simulink model "vit_tiny_simulink"  (R2026a)
settings: Solver=FixedStepAuto
values from neighbouring files (symbols this model uses):
  quantNet = quantize(quantObj)    [quantize_network.m]
libraries: dlconvfclib x26, dlnormalizationlib x25, dlcombinationlib x24, dlactivationlib x12
settings Model: Creator=arkadiyturevskiy  LastModifiedBy=arkadiyturevskiy
settings HardwareCC: ProdLargestAtomicInteger=Long  ProdLargestAtomicFloat=Double  ProdHWDeviceType=ARM Compatible->ARM Cortex-A
settings RTWCC: SystemTargetFile=ert.tlc  GenCodeOnly=on  GenerateReport=on  Description=Embedded Coder
settings ERTTargetCC: GenerateSampleERTMain=on

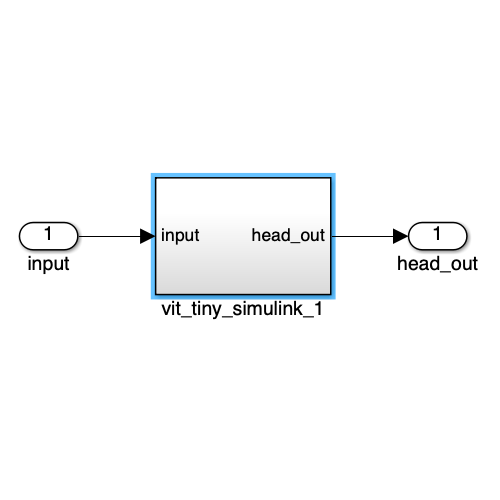
[thumbnail: Simulink's stored preview of the top-level diagram]
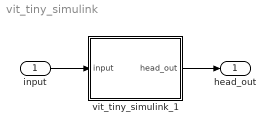
== system vit_tiny_simulink ==
  input : Inport  OutDataTypeStr=single  PortDimensions="[224  224    3]"
  vit_tiny_simulink_1 : Subsystem
  head_out : Outport
  wires:
  vit_tiny_simulink_1/1(head_out) -> head_out/1
  input/1 -> vit_tiny_simulink_1/1(input)

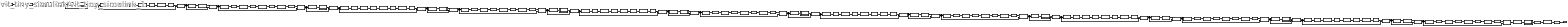
== system vit_tiny_simulink/vit_tiny_simulink_1 ==
  input : Inport  OutDataTypeStr=single  PortDimensions="[224  224    3]"
  block0_add1 : dlcombinationlib/Addition Layer  NumInputs=2  OutMin=[]  OutMax=[]  InternalRndMeth=Floor  InternalSaturateOnIntegerOverflow=off  SampleTime=-1
      settings: DataFormat=CT
  block0_add2 : dlcombinationlib/Addition Layer  NumInputs=2  OutMin=[]  OutMax=[]  InternalRndMeth=Floor  InternalSaturateOnIntegerOverflow=off  SampleTime=-1
      settings: DataFormat=CT
  block0_attn : Subsystem
  block0_fc1 : dlconvfclib/Fully Connected Layer  Layer=quantNet.Layers(10)  OutMin=[]  OutMax=[]  OutDataTypeStr=fixdt(1,32,9)  RndMeth=Nearest  WeightsDataTypeStr=fixdt(1,8,7)  WeightsMin=[]  WeightsMax=[]  BiasDataTypeStr=fixdt(1,32,9)  BiasMin=[]  BiasMax=[]  AccumDataTypeStr=fixdt(1,32,9)  AccumMin=[]  AccumMax=[]  InternalRndMeth=Nearest  InternalSaturateOnIntegerOverflow=off  SampleTime=-1
      settings: DataFormat=CT
  block0_fc1_in_cast : DataTypeConversion  OutDataTypeStr=fixdt(1,8,2)  RndMeth=Nearest
  block0_fc1_out_cast : DataTypeConversion  OutDataTypeStr=fixdt('single')  RndMeth=Nearest
  block0_fc2 : dlconvfclib/Fully Connected Layer  Layer=quantNet.Layers(12)  OutMin=[]  OutMax=[]  OutDataTypeStr=fixdt(1,32,9)  RndMeth=Nearest  WeightsDataTypeStr=fixdt(1,8,7)  WeightsMin=[]  WeightsMax=[]  BiasDataTypeStr=fixdt(1,32,9)  BiasMin=[]  BiasMax=[]  AccumDataTypeStr=fixdt(1,32,9)  AccumMin=[]  AccumMax=[]  InternalRndMeth=Nearest  InternalSaturateOnIntegerOverflow=off  SampleTime=-1
      settings: DataFormat=CT
  block0_fc2_in_cast : DataTypeConversion  OutDataTypeStr=fixdt(1,8,2)  RndMeth=Nearest
  block0_fc2_out_cast : DataTypeConversion  OutDataTypeStr=fixdt('single')  RndMeth=Nearest
  block0_gelu : dlactivationlib/GELU Layer  Approximation=none  OutMin=[]  OutMax=[]  SampleTime=-1
  block0_ln1 : dlnormalizationlib/Layer Normalization Layer  Layer=quantNet.Layers(6)  OutMin=[]  OutMax=[]  ScaleDataTypeStr=Inherit: Inherit via back propagation  ScaleMin=[]  ScaleMax=[]  OffsetDataTypeStr=Inherit: Inherit via back propagation  OffsetMin=[]  OffsetMax=[]  SampleTime=-1
      settings: DataFormat=CT
  block0_ln2 : dlnormalizationlib/Layer Normalization Layer  Layer=quantNet.Layers(9)  OutMin=[]  OutMax=[]  ScaleDataTypeStr=Inherit: Inherit via back propagation  ScaleMin=[]  ScaleMax=[]  OffsetDataTypeStr=Inherit: Inherit via back propagation  OffsetMin=[]  OffsetMax=[]  SampleTime=-1
      settings: DataFormat=CT
  block10_add1 : dlcombinationlib/Addition Layer  NumInputs=2  OutMin=[]  OutMax=[]  InternalRndMeth=Floor  InternalSaturateOnIntegerOverflow=off  SampleTime=-1
      settings: DataFormat=CT
  block10_add2 : dlcombinationlib/Addition Layer  NumInputs=2  OutMin=[]  OutMax=[]  InternalRndMeth=Floor  InternalSaturateOnIntegerOverflow=off  SampleTime=-1
      settings: DataFormat=CT
  block10_attn : Subsystem
  block10_fc1 : dlconvfclib/Fully Connected Layer  Layer=quantNet.Layers(90)  OutMin=[]  OutMax=[]  OutDataTypeStr=fixdt(1,32,10)  RndMeth=Nearest  WeightsDataTypeStr=fixdt(1,8,7)  WeightsMin=[]  WeightsMax=[]  BiasDataTypeStr=fixdt(1,32,10)  BiasMin=[]  BiasMax=[]  AccumDataTypeStr=fixdt(1,32,10)  AccumMin=[]  AccumMax=[]  InternalRndMeth=Nearest  InternalSaturateOnIntegerOverflow=off  SampleTime=-1
      settings: DataFormat=CT
  block10_fc1_in_cast : DataTypeConversion  OutDataTypeStr=fixdt(1,8,3)  RndMeth=Nearest
  block10_fc1_out_cast : DataTypeConversion  OutDataTypeStr=fixdt('single')  RndMeth=Nearest
  block10_fc2 : dlconvfclib/Fully Connected Layer  Layer=quantNet.Layers(92)  OutMin=[]  OutMax=[]  OutDataTypeStr=fixdt(1,32,11)  RndMeth=Nearest  WeightsDataTypeStr=fixdt(1,8,7)  WeightsMin=[]  WeightsMax=[]  BiasDataTypeStr=fixdt(1,32,11)  BiasMin=[]  BiasMax=[]  AccumDataTypeStr=fixdt(1,32,11)  AccumMin=[]  AccumMax=[]  InternalRndMeth=Nearest  InternalSaturateOnIntegerOverflow=off  SampleTime=-1
      settings: DataFormat=CT
  block10_fc2_in_cast : DataTypeConversion  OutDataTypeStr=fixdt(1,8,4)  RndMeth=Nearest
  block10_fc2_out_cast : DataTypeConversion  OutDataTypeStr=fixdt('single')  RndMeth=Nearest
  block10_gelu : dlactivationlib/GELU Layer  Approximation=none  OutMin=[]  OutMax=[]  SampleTime=-1
  block10_ln1 : dlnormalizationlib/Layer Normalization Layer  Layer=quantNet.Layers(86)  OutMin=[]  OutMax=[]  ScaleDataTypeStr=Inherit: Inherit via back propagation  ScaleMin=[]  ScaleMax=[]  OffsetDataTypeStr=Inherit: Inherit via back propagation  OffsetMin=[]  OffsetMax=[]  SampleTime=-1
      settings: DataFormat=CT
  block10_ln2 : dlnormalizationlib/Layer Normalization Layer  Layer=quantNet.Layers(89)  OutMin=[]  OutMax=[]  ScaleDataTypeStr=Inherit: Inherit via back propagation  ScaleMin=[]  ScaleMax=[]  OffsetDataTypeStr=Inherit: Inherit via back propagation  OffsetMin=[]  OffsetMax=[]  SampleTime=-1
      settings: DataFormat=CT
  block11_add1 : dlcombinationlib/Addition Layer  NumInputs=2  OutMin=[]  OutMax=[]  InternalRndMeth=Floor  InternalSaturateOnIntegerOverflow=off  SampleTime=-1
      settings: DataFormat=CT
  block11_add2 : dlcombinationlib/Addition Layer  NumInputs=2  OutMin=[]  OutMax=[]  InternalRndMeth=Floor  InternalSaturateOnIntegerOverflow=off  SampleTime=-1
      settings: DataFormat=CT
  block11_attn : Subsystem
  block11_fc1 : dlconvfclib/Fully Connected Layer  Layer=quantNet.Layers(98)  OutMin=[]  OutMax=[]  OutDataTypeStr=fixdt(1,32,11)  RndMeth=Nearest  WeightsDataTypeStr=fixdt(1,8,8)  WeightsMin=[]  WeightsMax=[]  BiasDataTypeStr=fixdt(1,32,11)  BiasMin=[]  BiasMax=[]  AccumDataTypeStr=fixdt(1,32,11)  AccumMin=[]  AccumMax=[]  InternalRndMeth=Nearest  InternalSaturateOnIntegerOverflow=off  SampleTime=-1
      settings: DataFormat=CT
  block11_fc1_in_cast : DataTypeConversion  OutDataTypeStr=fixdt(1,8,3)  RndMeth=Nearest
  block11_fc1_out_cast : DataTypeConversion  OutDataTypeStr=fixdt('single')  RndMeth=Nearest
  block11_fc2 : dlconvfclib/Fully Connected Layer  Layer=quantNet.Layers(100)  OutMin=[]  OutMax=[]  OutDataTypeStr=fixdt(1,32,11)  RndMeth=Nearest  WeightsDataTypeStr=fixdt(1,8,7)  WeightsMin=[]  WeightsMax=[]  BiasDataTypeStr=fixdt(1,32,11)  BiasMin=[]  BiasMax=[]  AccumDataTypeStr=fixdt(1,32,11)  AccumMin=[]  AccumMax=[]  InternalRndMeth=Nearest  InternalSaturateOnIntegerOverflow=off  SampleTime=-1
      settings: DataFormat=CT
  block11_fc2_in_cast : DataTypeConversion  OutDataTypeStr=fixdt(1,8,4)  RndMeth=Nearest
  block11_fc2_out_cast : DataTypeConversion  OutDataTypeStr=fixdt('single')  RndMeth=Nearest
  block11_gelu : dlactivationlib/GELU Layer  Approximation=none  OutMin=[]  OutMax=[]  SampleTime=-1
  block11_ln1 : dlnormalizationlib/Layer Normalization Layer  Layer=quantNet.Layers(94)  OutMin=[]  OutMax=[]  ScaleDataTypeStr=Inherit: Inherit via back propagation  ScaleMin=[]  ScaleMax=[]  OffsetDataTypeStr=Inherit: Inherit via back propagation  OffsetMin=[]  OffsetMax=[]  SampleTime=-1
      settings: DataFormat=CT
  block11_ln2 : dlnormalizationlib/Layer Normalization Layer  Layer=quantNet.Layers(97)  OutMin=[]  OutMax=[]  ScaleDataTypeStr=Inherit: Inherit via back propagation  ScaleMin=[]  ScaleMax=[]  OffsetDataTypeStr=Inherit: Inherit via back propagation  OffsetMin=[]  OffsetMax=[]  SampleTime=-1
      settings: DataFormat=CT
  block1_add1 : dlcombinationlib/Addition Layer  NumInputs=2  OutMin=[]  OutMax=[]  InternalRndMeth=Floor  InternalSaturateOnIntegerOverflow=off  SampleTime=-1
      settings: DataFormat=CT
  block1_add2 : dlcombinationlib/Addition Layer  NumInputs=2  OutMin=[]  OutMax=[]  InternalRndMeth=Floor  InternalSaturateOnIntegerOverflow=off  SampleTime=-1
      settings: DataFormat=CT
  block1_attn : Subsystem
  block1_fc1 : dlconvfclib/Fully Connected Layer  Layer=quantNet.Layers(18)  OutMin=[]  OutMax=[]  OutDataTypeStr=fixdt(1,32,10)  RndMeth=Nearest  WeightsDataTypeStr=fixdt(1,8,7)  WeightsMin=[]  WeightsMax=[]  BiasDataTypeStr=fixdt(1,32,10)  BiasMin=[]  BiasMax=[]  AccumDataTypeStr=fixdt(1,32,10)  AccumMin=[]  AccumMax=[]  InternalRndMeth=Nearest  InternalSaturateOnIntegerOverflow=off  SampleTime=-1
      settings: DataFormat=CT
  block1_fc1_in_cast : DataTypeConversion  OutDataTypeStr=fixdt(1,8,3)  RndMeth=Nearest
  block1_fc1_out_cast : DataTypeConversion  OutDataTypeStr=fixdt('single')  RndMeth=Nearest
  block1_fc2 : dlconvfclib/Fully Connected Layer  Layer=quantNet.Layers(20)  OutMin=[]  OutMax=[]  OutDataTypeStr=fixdt(1,32,10)  RndMeth=Nearest  WeightsDataTypeStr=fixdt(1,8,7)  WeightsMin=[]  WeightsMax=[]  BiasDataTypeStr=fixdt(1,32,10)  BiasMin=[]  BiasMax=[]  AccumDataTypeStr=fixdt(1,32,10)  AccumMin=[]  AccumMax=[]  InternalRndMeth=Nearest  InternalSaturateOnIntegerOverflow=off  SampleTime=-1
      settings: DataFormat=CT
  block1_fc2_in_cast : DataTypeConversion  OutDataTypeStr=fixdt(1,8,3)  RndMeth=Nearest
  block1_fc2_out_cast : DataTypeConversion  OutDataTypeStr=fixdt('single')  RndMeth=Nearest
  block1_gelu : dlactivationlib/GELU Layer  Approximation=none  OutMin=[]  OutMax=[]  SampleTime=-1
  block1_ln1 : dlnormalizationlib/Layer Normalization Layer  Layer=quantNet.Layers(14)  OutMin=[]  OutMax=[]  ScaleDataTypeStr=Inherit: Inherit via back propagation  ScaleMin=[]  ScaleMax=[]  OffsetDataTypeStr=Inherit: Inherit via back propagation  OffsetMin=[]  OffsetMax=[]  SampleTime=-1
      settings: DataFormat=CT
  block1_ln2 : dlnormalizationlib/Layer Normalization Layer  Layer=quantNet.Layers(17)  OutMin=[]  OutMax=[]  ScaleDataTypeStr=Inherit: Inherit via back propagation  ScaleMin=[]  ScaleMax=[]  OffsetDataTypeStr=Inherit: Inherit via back propagation  OffsetMin=[]  OffsetMax=[]  SampleTime=-1
      settings: DataFormat=CT
  block2_add1 : dlcombinationlib/Addition Layer  NumInputs=2  OutMin=[]  OutMax=[]  InternalRndMeth=Floor  InternalSaturateOnIntegerOverflow=off  SampleTime=-1
      settings: DataFormat=CT
  block2_add2 : dlcombinationlib/Addition Layer  NumInputs=2  OutMin=[]  OutMax=[]  InternalRndMeth=Floor  InternalSaturateOnIntegerOverflow=off  SampleTime=-1
      settings: DataFormat=CT
  block2_attn : Subsystem
  block2_fc1 : dlconvfclib/Fully Connected Layer  Layer=quantNet.Layers(26)  OutMin=[]  OutMax=[]  OutDataTypeStr=fixdt(1,32,10)  RndMeth=Nearest  WeightsDataTypeStr=fixdt(1,8,7)  WeightsMin=[]  WeightsMax=[]  BiasDataTypeStr=fixdt(1,32,10)  BiasMin=[]  BiasMax=[]  AccumDataTypeStr=fixdt(1,32,10)  AccumMin=[]  AccumMax=[]  InternalRndMeth=Nearest  InternalSaturateOnIntegerOverflow=off  SampleTime=-1
      settings: DataFormat=CT
  block2_fc1_in_cast : DataTypeConversion  OutDataTypeStr=fixdt(1,8,3)  RndMeth=Nearest
  block2_fc1_out_cast : DataTypeConversion  OutDataTypeStr=fixdt('single')  RndMeth=Nearest
  block2_fc2 : dlconvfclib/Fully Connected Layer  Layer=quantNet.Layers(28)  OutMin=[]  OutMax=[]  OutDataTypeStr=fixdt(1,32,10)  RndMeth=Nearest  WeightsDataTypeStr=fixdt(1,8,7)  WeightsMin=[]  WeightsMax=[]  BiasDataTypeStr=fixdt(1,32,10)  BiasMin=[]  BiasMax=[]  AccumDataTypeStr=fixdt(1,32,10)  AccumMin=[]  AccumMax=[]  InternalRndMeth=Nearest  InternalSaturateOnIntegerOverflow=off  SampleTime=-1
      settings: DataFormat=CT
  block2_fc2_in_cast : DataTypeConversion  OutDataTypeStr=fixdt(1,8,3)  RndMeth=Nearest
  block2_fc2_out_cast : DataTypeConversion  OutDataTypeStr=fixdt('single')  RndMeth=Nearest
  block2_gelu : dlactivationlib/GELU Layer  Approximation=none  OutMin=[]  OutMax=[]  SampleTime=-1
  block2_ln1 : dlnormalizationlib/Layer Normalization Layer  Layer=quantNet.Layers(22)  OutMin=[]  OutMax=[]  ScaleDataTypeStr=Inherit: Inherit via back propagation  ScaleMin=[]  ScaleMax=[]  OffsetDataTypeStr=Inherit: Inherit via back propagation  OffsetMin=[]  OffsetMax=[]  SampleTime=-1
      settings: DataFormat=CT
  block2_ln2 : dlnormalizationlib/Layer Normalization Layer  Layer=quantNet.Layers(25)  OutMin=[]  OutMax=[]  ScaleDataTypeStr=Inherit: Inherit via back propagation  ScaleMin=[]  ScaleMax=[]  OffsetDataTypeStr=Inherit: Inherit via back propagation  OffsetMin=[]  OffsetMax=[]  SampleTime=-1
      settings: DataFormat=CT
  block3_add1 : dlcombinationlib/Addition Layer  NumInputs=2  OutMin=[]  OutMax=[]  InternalRndMeth=Floor  InternalSaturateOnIntegerOverflow=off  SampleTime=-1
      settings: DataFormat=CT
  block3_add2 : dlcombinationlib/Addition Layer  NumInputs=2  OutMin=[]  OutMax=[]  InternalRndMeth=Floor  InternalSaturateOnIntegerOverflow=off  SampleTime=-1
      settings: DataFormat=CT
  block3_attn : Subsystem
  block3_fc1 : dlconvfclib/Fully Connected Layer  Layer=quantNet.Layers(34)  OutMin=[]  OutMax=[]  OutDataTypeStr=fixdt(1,32,10)  RndMeth=Nearest  WeightsDataTypeStr=fixdt(1,8,7)  WeightsMin=[]  WeightsMax=[]  BiasDataTypeStr=fixdt(1,32,10)  BiasMin=[]  BiasMax=[]  AccumDataTypeStr=fixdt(1,32,10)  AccumMin=[]  AccumMax=[]  InternalRndMeth=Nearest  InternalSaturateOnIntegerOverflow=off  SampleTime=-1
      settings: DataFormat=CT
  block3_fc1_in_cast : DataTypeConversion  OutDataTypeStr=fixdt(1,8,3)  RndMeth=Nearest
  block3_fc1_out_cast : DataTypeConversion  OutDataTypeStr=fixdt('single')  RndMeth=Nearest
  block3_fc2 : dlconvfclib/Fully Connected Layer  Layer=quantNet.Layers(36)  OutMin=[]  OutMax=[]  OutDataTypeStr=fixdt(1,32,11)  RndMeth=Nearest  WeightsDataTypeStr=fixdt(1,8,7)  WeightsMin=[]  WeightsMax=[]  BiasDataTypeStr=fixdt(1,32,11)  BiasMin=[]  BiasMax=[]  AccumDataTypeStr=fixdt(1,32,11)  AccumMin=[]  AccumMax=[]  InternalRndMeth=Nearest  InternalSaturateOnIntegerOverflow=off  SampleTime=-1
      settings: DataFormat=CT
  block3_fc2_in_cast : DataTypeConversion  OutDataTypeStr=fixdt(1,8,4)  RndMeth=Nearest
  block3_fc2_out_cast : DataTypeConversion  OutDataTypeStr=fixdt('single')  RndMeth=Nearest
  block3_gelu : dlactivationlib/GELU Layer  Approximation=none  OutMin=[]  OutMax=[]  SampleTime=-1
  block3_ln1 : dlnormalizationlib/Layer Normalization Layer  Layer=quantNet.Layers(30)  OutMin=[]  OutMax=[]  ScaleDataTypeStr=Inherit: Inherit via back propagation  ScaleMin=[]  ScaleMax=[]  OffsetDataTypeStr=Inherit: Inherit via back propagation  OffsetMin=[]  OffsetMax=[]  SampleTime=-1
      settings: DataFormat=CT
  block3_ln2 : dlnormalizationlib/Layer Normalization Layer  Layer=quantNet.Layers(33)  OutMin=[]  OutMax=[]  ScaleDataTypeStr=Inherit: Inherit via back propagation  ScaleMin=[]  ScaleMax=[]  OffsetDataTypeStr=Inherit: Inherit via back propagation  OffsetMin=[]  OffsetMax=[]  SampleTime=-1
      settings: DataFormat=CT
  block4_add1 : dlcombinationlib/Addition Layer  NumInputs=2  OutMin=[]  OutMax=[]  InternalRndMeth=Floor  InternalSaturateOnIntegerOverflow=off  SampleTime=-1
      settings: DataFormat=CT
  block4_add2 : dlcombinationlib/Addition Layer  NumInputs=2  OutMin=[]  OutMax=[]  InternalRndMeth=Floor  InternalSaturateOnIntegerOverflow=off  SampleTime=-1
      settings: DataFormat=CT
  block4_attn : Subsystem
  block4_fc1 : dlconvfclib/Fully Connected Layer  Layer=quantNet.Layers(42)  OutMin=[]  OutMax=[]  OutDataTypeStr=fixdt(1,32,12)  RndMeth=Nearest  WeightsDataTypeStr=fixdt(1,8,8)  WeightsMin=[]  WeightsMax=[]  BiasDataTypeStr=fixdt(1,32,12)  BiasMin=[]  BiasMax=[]  AccumDataTypeStr=fixdt(1,32,12)  AccumMin=[]  AccumMax=[]  InternalRndMeth=Nearest  InternalSaturateOnIntegerOverflow=off  SampleTime=-1
      settings: DataFormat=CT
  block4_fc1_in_cast : DataTypeConversion  OutDataTypeStr=fixdt(1,8,4)  RndMeth=Nearest
  block4_fc1_out_cast : DataTypeConversion  OutDataTypeStr=fixdt('single')  RndMeth=Nearest
  block4_fc2 : dlconvfclib/Fully Connected Layer  Layer=quantNet.Layers(44)  OutMin=[]  OutMax=[]  OutDataTypeStr=fixdt(1,32,12)  RndMeth=Nearest  WeightsDataTypeStr=fixdt(1,8,8)  WeightsMin=[]  WeightsMax=[]  BiasDataTypeStr=fixdt(1,32,12)  BiasMin=[]  BiasMax=[]  AccumDataTypeStr=fixdt(1,32,12)  AccumMin=[]  AccumMax=[]  InternalRndMeth=Nearest  InternalSaturateOnIntegerOverflow=off  SampleTime=-1
      settings: DataFormat=CT
  block4_fc2_in_cast : DataTypeConversion  OutDataTypeStr=fixdt(1,8,4)  RndMeth=Nearest
  block4_fc2_out_cast : DataTypeConversion  OutDataTypeStr=fixdt('single')  RndMeth=Nearest
  block4_gelu : dlactivationlib/GELU Layer  Approximation=none  OutMin=[]  OutMax=[]  SampleTime=-1
  block4_ln1 : dlnormalizationlib/Layer Normalization Layer  Layer=quantNet.Layers(38)  OutMin=[]  OutMax=[]  ScaleDataTypeStr=Inherit: Inherit via back propagation  ScaleMin=[]  ScaleMax=[]  OffsetDataTypeStr=Inherit: Inherit via back propagation  OffsetMin=[]  OffsetMax=[]  SampleTime=-1
      settings: DataFormat=CT
  block4_ln2 : dlnormalizationlib/Layer Normalization Layer  Layer=quantNet.Layers(41)  OutMin=[]  OutMax=[]  ScaleDataTypeStr=Inherit: Inherit via back propagation  ScaleMin=[]  ScaleMax=[]  OffsetDataTypeStr=Inherit: Inherit via back propagation  OffsetMin=[]  OffsetMax=[]  SampleTime=-1
      settings: DataFormat=CT
  block5_add1 : dlcombinationlib/Addition Layer  NumInputs=2  OutMin=[]  OutMax=[]  InternalRndMeth=Floor  InternalSaturateOnIntegerOverflow=off  SampleTime=-1
      settings: DataFormat=CT
  block5_add2 : dlcombinationlib/Addition Layer  NumInputs=2  OutMin=[]  OutMax=[]  InternalRndMeth=Floor  InternalSaturateOnIntegerOverflow=off  SampleTime=-1
      settings: DataFormat=CT
  block5_attn : Subsystem
  block5_fc1 : dlconvfclib/Fully Connected Layer  Layer=quantNet.Layers(50)  OutMin=[]  OutMax=[]  OutDataTypeStr=fixdt(1,32,12)  RndMeth=Nearest  WeightsDataTypeStr=fixdt(1,8,8)  WeightsMin=[]  WeightsMax=[]  BiasDataTypeStr=fixdt(1,32,12)  BiasMin=[]  BiasMax=[]  AccumDataTypeStr=fixdt(1,32,12)  AccumMin=[]  AccumMax=[]  InternalRndMeth=Nearest  InternalSaturateOnIntegerOverflow=off  SampleTime=-1
      settings: DataFormat=CT
  block5_fc1_in_cast : DataTypeConversion  OutDataTypeStr=fixdt(1,8,4)  RndMeth=Nearest
  block5_fc1_out_cast : DataTypeConversion  OutDataTypeStr=fixdt('single')  RndMeth=Nearest
  block5_fc2 : dlconvfclib/Fully Connected Layer  Layer=quantNet.Layers(52)  OutMin=[]  OutMax=[]  OutDataTypeStr=fixdt(1,32,12)  RndMeth=Nearest  WeightsDataTypeStr=fixdt(1,8,8)  WeightsMin=[]  WeightsMax=[]  BiasDataTypeStr=fixdt(1,32,12)  BiasMin=[]  BiasMax=[]  AccumDataTypeStr=fixdt(1,32,12)  AccumMin=[]  AccumMax=[]  InternalRndMeth=Nearest  InternalSaturateOnIntegerOverflow=off  SampleTime=-1
      settings: DataFormat=CT
  block5_fc2_in_cast : DataTypeConversion  OutDataTypeStr=fixdt(1,8,4)  RndMeth=Nearest
  block5_fc2_out_cast : DataTypeConversion  OutDataTypeStr=fixdt('single')  RndMeth=Nearest
  block5_gelu : dlactivationlib/GELU Layer  Approximation=none  OutMin=[]  OutMax=[]  SampleTime=-1
  block5_ln1 : dlnormalizationlib/Layer Normalization Layer  Layer=quantNet.Layers(46)  OutMin=[]  OutMax=[]  ScaleDataTypeStr=Inherit: Inherit via back propagation  ScaleMin=[]  ScaleMax=[]  OffsetDataTypeStr=Inherit: Inherit via back propagation  OffsetMin=[]  OffsetMax=[]  SampleTime=-1
      settings: DataFormat=CT
  block5_ln2 : dlnormalizationlib/Layer Normalization Layer  Layer=quantNet.Layers(49)  OutMin=[]  OutMax=[]  ScaleDataTypeStr=Inherit: Inherit via back propagation  ScaleMin=[]  ScaleMax=[]  OffsetDataTypeStr=Inherit: Inherit via back propagation  OffsetMin=[]  OffsetMax=[]  SampleTime=-1
      settings: DataFormat=CT
  block6_add1 : dlcombinationlib/Addition Layer  NumInputs=2  OutMin=[]  OutMax=[]  InternalRndMeth=Floor  InternalSaturateOnIntegerOverflow=off  SampleTime=-1
      settings: DataFormat=CT
  block6_add2 : dlcombinationlib/Addition Layer  NumInputs=2  OutMin=[]  OutMax=[]  InternalRndMeth=Floor  InternalSaturateOnIntegerOverflow=off  SampleTime=-1
      settings: DataFormat=CT
  block6_attn : Subsystem
  block6_fc1 : dlconvfclib/Fully Connected Layer  Layer=quantNet.Layers(58)  OutMin=[]  OutMax=[]  OutDataTypeStr=fixdt(1,32,12)  RndMeth=Nearest  WeightsDataTypeStr=fixdt(1,8,8)  WeightsMin=[]  WeightsMax=[]  BiasDataTypeStr=fixdt(1,32,12)  BiasMin=[]  BiasMax=[]  AccumDataTypeStr=fixdt(1,32,12)  AccumMin=[]  AccumMax=[]  InternalRndMeth=Nearest  InternalSaturateOnIntegerOverflow=off  SampleTime=-1
      settings: DataFormat=CT
  block6_fc1_in_cast : DataTypeConversion  OutDataTypeStr=fixdt(1,8,4)  RndMeth=Nearest
  block6_fc1_out_cast : DataTypeConversion  OutDataTypeStr=fixdt('single')  RndMeth=Nearest
  block6_fc2 : dlconvfclib/Fully Connected Layer  Layer=quantNet.Layers(60)  OutMin=[]  OutMax=[]  OutDataTypeStr=fixdt(1,32,10)  RndMeth=Nearest  WeightsDataTypeStr=fixdt(1,8,7)  WeightsMin=[]  WeightsMax=[]  BiasDataTypeStr=fixdt(1,32,10)  BiasMin=[]  BiasMax=[]  AccumDataTypeStr=fixdt(1,32,10)  AccumMin=[]  AccumMax=[]  InternalRndMeth=Nearest  InternalSaturateOnIntegerOverflow=off  SampleTime=-1
      settings: DataFormat=CT
  block6_fc2_in_cast : DataTypeConversion  OutDataTypeStr=fixdt(1,8,3)  RndMeth=Nearest
  block6_fc2_out_cast : DataTypeConversion  OutDataTypeStr=fixdt('single')  RndMeth=Nearest
  block6_gelu : dlactivationlib/GELU Layer  Approximation=none  OutMin=[]  OutMax=[]  SampleTime=-1
  block6_ln1 : dlnormalizationlib/Layer Normalization Layer  Layer=quantNet.Layers(54)  OutMin=[]  OutMax=[]  ScaleDataTypeStr=Inherit: Inherit via back propagation  ScaleMin=[]  ScaleMax=[]  OffsetDataTypeStr=Inherit: Inherit via back propagation  OffsetMin=[]  OffsetMax=[]  SampleTime=-1
      settings: DataFormat=CT
  block6_ln2 : dlnormalizationlib/Layer Normalization Layer  Layer=quantNet.Layers(57)  OutMin=[]  OutMax=[]  ScaleDataTypeStr=Inherit: Inherit via back propagation  ScaleMin=[]  ScaleMax=[]  OffsetDataTypeStr=Inherit: Inherit via back propagation  OffsetMin=[]  OffsetMax=[]  SampleTime=-1
      settings: DataFormat=CT
  block7_add1 : dlcombinationlib/Addition Layer  NumInputs=2  OutMin=[]  OutMax=[]  InternalRndMeth=Floor  InternalSaturateOnIntegerOverflow=off  SampleTime=-1
      settings: DataFormat=CT
  block7_add2 : dlcombinationlib/Addition Layer  NumInputs=2  OutMin=[]  OutMax=[]  InternalRndMeth=Floor  InternalSaturateOnIntegerOverflow=off  SampleTime=-1
      settings: DataFormat=CT
  block7_attn : Subsystem
  block7_fc1 : dlconvfclib/Fully Connected Layer  Layer=quantNet.Layers(66)  OutMin=[]  OutMax=[]  OutDataTypeStr=fixdt(1,32,9)  RndMeth=Nearest  WeightsDataTypeStr=fixdt(1,8,5)  WeightsMin=[]  WeightsMax=[]  BiasDataTypeStr=fixdt(1,32,9)  BiasMin=[]  BiasMax=[]  AccumDataTypeStr=fixdt(1,32,9)  AccumMin=[]  AccumMax=[]  InternalRndMeth=Nearest  InternalSaturateOnIntegerOverflow=off  SampleTime=-1
      settings: DataFormat=CT
  block7_fc1_in_cast : DataTypeConversion  OutDataTypeStr=fixdt(1,8,4)  RndMeth=Nearest
  block7_fc1_out_cast : DataTypeConversion  OutDataTypeStr=fixdt('single')  RndMeth=Nearest
  block7_fc2 : dlconvfclib/Fully Connected Layer  Layer=quantNet.Layers(68)  OutMin=[]  OutMax=[]  OutDataTypeStr=fixdt(1,32,4)  RndMeth=Nearest  WeightsDataTypeStr=fixdt(1,8,5)  WeightsMin=[]  WeightsMax=[]  BiasDataTypeStr=fixdt(1,32,4)  BiasMin=[]  BiasMax=[]  AccumDataTypeStr=fixdt(1,32,4)  AccumMin=[]  AccumMax=[]  InternalRndMeth=Nearest  InternalSaturateOnIntegerOverflow=off  SampleTime=-1
      settings: DataFormat=CT
  block7_fc2_in_cast : DataTypeConversion  OutDataTypeStr=fixdt(1,8,-1)  RndMeth=Nearest
  block7_fc2_out_cast : DataTypeConversion  OutDataTypeStr=fixdt('single')  RndMeth=Nearest
  block7_gelu : dlactivationlib/GELU Layer  Approximation=none  OutMin=[]  OutMax=[]  SampleTime=-1
  block7_ln1 : dlnormalizationlib/Layer Normalization Layer  Layer=quantNet.Layers(62)  OutMin=[]  OutMax=[]  ScaleDataTypeStr=Inherit: Inherit via back propagation  ScaleMin=[]  ScaleMax=[]  OffsetDataTypeStr=Inherit: Inherit via back propagation  OffsetMin=[]  OffsetMax=[]  SampleTime=-1
      settings: DataFormat=CT
  block7_ln2 : dlnormalizationlib/Layer Normalization Layer  Layer=quantNet.Layers(65)  OutMin=[]  OutMax=[]  ScaleDataTypeStr=Inherit: Inherit via back propagation  ScaleMin=[]  ScaleMax=[]  OffsetDataTypeStr=Inherit: Inherit via back propagation  OffsetMin=[]  OffsetMax=[]  SampleTime=-1
      settings: DataFormat=CT
  block8_add1 : dlcombinationlib/Addition Layer  NumInputs=2  OutMin=[]  OutMax=[]  InternalRndMeth=Floor  InternalSaturateOnIntegerOverflow=off  SampleTime=-1
      settings: DataFormat=CT
  block8_add2 : dlcombinationlib/Addition Layer  NumInputs=2  OutMin=[]  OutMax=[]  InternalRndMeth=Floor  InternalSaturateOnIntegerOverflow=off  SampleTime=-1
      settings: DataFormat=CT
  block8_attn : Subsystem
  block8_fc1 : dlconvfclib/Fully Connected Layer  Layer=quantNet.Layers(74)  OutMin=[]  OutMax=[]  OutDataTypeStr=fixdt(1,32,11)  RndMeth=Nearest  WeightsDataTypeStr=fixdt(1,8,8)  WeightsMin=[]  WeightsMax=[]  BiasDataTypeStr=fixdt(1,32,11)  BiasMin=[]  BiasMax=[]  AccumDataTypeStr=fixdt(1,32,11)  AccumMin=[]  AccumMax=[]  InternalRndMeth=Nearest  InternalSaturateOnIntegerOverflow=off  SampleTime=-1
      settings: DataFormat=CT
  block8_fc1_in_cast : DataTypeConversion  OutDataTypeStr=fixdt(1,8,3)  RndMeth=Nearest
  block8_fc1_out_cast : DataTypeConversion  OutDataTypeStr=fixdt('single')  RndMeth=Nearest
  block8_fc2 : dlconvfclib/Fully Connected Layer  Layer=quantNet.Layers(76)  OutMin=[]  OutMax=[]  OutDataTypeStr=fixdt(1,32,11)  RndMeth=Nearest  WeightsDataTypeStr=fixdt(1,8,7)  WeightsMin=[]  WeightsMax=[]  BiasDataTypeStr=fixdt(1,32,11)  BiasMin=[]  BiasMax=[]  AccumDataTypeStr=fixdt(1,32,11)  AccumMin=[]  AccumMax=[]  InternalRndMeth=Nearest  InternalSaturateOnIntegerOverflow=off  SampleTime=-1
      settings: DataFormat=CT
  block8_fc2_in_cast : DataTypeConversion  OutDataTypeStr=fixdt(1,8,4)  RndMeth=Nearest
  block8_fc2_out_cast : DataTypeConversion  OutDataTypeStr=fixdt('single')  RndMeth=Nearest
  block8_gelu : dlactivationlib/GELU Layer  Approximation=none  OutMin=[]  OutMax=[]  SampleTime=-1
  block8_ln1 : dlnormalizationlib/Layer Normalization Layer  Layer=quantNet.Layers(70)  OutMin=[]  OutMax=[]  ScaleDataTypeStr=Inherit: Inherit via back propagation  ScaleMin=[]  ScaleMax=[]  OffsetDataTypeStr=Inherit: Inherit via back propagation  OffsetMin=[]  OffsetMax=[]  SampleTime=-1
      settings: DataFormat=CT
  block8_ln2 : dlnormalizationlib/Layer Normalization Layer  Layer=quantNet.Layers(73)  OutMin=[]  OutMax=[]  ScaleDataTypeStr=Inherit: Inherit via back propagation  ScaleMin=[]  ScaleMax=[]  OffsetDataTypeStr=Inherit: Inherit via back propagation  OffsetMin=[]  OffsetMax=[]  SampleTime=-1
      settings: DataFormat=CT
  block9_add1 : dlcombinationlib/Addition Layer  NumInputs=2  OutMin=[]  OutMax=[]  InternalRndMeth=Floor  InternalSaturateOnIntegerOverflow=off  SampleTime=-1
      settings: DataFormat=CT
  block9_add2 : dlcombinationlib/Addition Layer  NumInputs=2  OutMin=[]  OutMax=[]  InternalRndMeth=Floor  InternalSaturateOnIntegerOverflow=off  SampleTime=-1
      settings: DataFormat=CT
  block9_attn : Subsystem
  block9_fc1 : dlconvfclib/Fully Connected Layer  Layer=quantNet.Layers(82)  OutMin=[]  OutMax=[]  OutDataTypeStr=fixdt(1,32,10)  RndMeth=Nearest  WeightsDataTypeStr=fixdt(1,8,7)  WeightsMin=[]  WeightsMax=[]  BiasDataTypeStr=fixdt(1,32,10)  BiasMin=[]  BiasMax=[]  AccumDataTypeStr=fixdt(1,32,10)  AccumMin=[]  AccumMax=[]  InternalRndMeth=Nearest  InternalSaturateOnIntegerOverflow=off  SampleTime=-1
      settings: DataFormat=CT
  block9_fc1_in_cast : DataTypeConversion  OutDataTypeStr=fixdt(1,8,3)  RndMeth=Nearest
  block9_fc1_out_cast : DataTypeConversion  OutDataTypeStr=fixdt('single')  RndMeth=Nearest
  block9_fc2 : dlconvfclib/Fully Connected Layer  Layer=quantNet.Layers(84)  OutMin=[]  OutMax=[]  OutDataTypeStr=fixdt(1,32,11)  RndMeth=Nearest  WeightsDataTypeStr=fixdt(1,8,7)  WeightsMin=[]  WeightsMax=[]  BiasDataTypeStr=fixdt(1,32,11)  BiasMin=[]  BiasMax=[]  AccumDataTypeStr=fixdt(1,32,11)  AccumMin=[]  AccumMax=[]  InternalRndMeth=Nearest  InternalSaturateOnIntegerOverflow=off  SampleTime=-1
      settings: DataFormat=CT
  block9_fc2_in_cast : DataTypeConversion  OutDataTypeStr=fixdt(1,8,4)  RndMeth=Nearest
  block9_fc2_out_cast : DataTypeConversion  OutDataTypeStr=fixdt('single')  RndMeth=Nearest
  block9_gelu : dlactivationlib/GELU Layer  Approximation=none  OutMin=[]  OutMax=[]  SampleTime=-1
  block9_ln1 : dlnormalizationlib/Layer Normalization Layer  Layer=quantNet.Layers(78)  OutMin=[]  OutMax=[]  ScaleDataTypeStr=Inherit: Inherit via back propagation  ScaleMin=[]  ScaleMax=[]  OffsetDataTypeStr=Inherit: Inherit via back propagation  OffsetMin=[]  OffsetMax=[]  SampleTime=-1
      settings: DataFormat=CT
  block9_ln2 : dlnormalizationlib/Layer Normalization Layer  Layer=quantNet.Layers(81)  OutMin=[]  OutMax=[]  ScaleDataTypeStr=Inherit: Inherit via back propagation  ScaleMin=[]  ScaleMax=[]  OffsetDataTypeStr=Inherit: Inherit via back propagation  OffsetMin=[]  OffsetMax=[]  SampleTime=-1
      settings: DataFormat=CT
  cls_extract : Subsystem
  cls_prepend : Subsystem
  final_ln : dlnormalizationlib/Layer Normalization Layer  Layer=quantNet.Layers(102)  OutMin=[]  OutMax=[]  ScaleDataTypeStr=Inherit: Inherit via back propagation  ScaleMin=[]  ScaleMax=[]  OffsetDataTypeStr=Inherit: Inherit via back propagation  OffsetMin=[]  OffsetMax=[]  SampleTime=-1
      settings: DataFormat=CT
  head : dlconvfclib/Fully Connected Layer  Layer=quantNet.Layers(104)  OutMin=[]  OutMax=[]  OutDataTypeStr=fixdt(1,32,11)  RndMeth=Nearest  WeightsDataTypeStr=fixdt(1,8,9)  WeightsMin=[]  WeightsMax=[]  BiasDataTypeStr=fixdt(1,32,11)  BiasMin=[]  BiasMax=[]  AccumDataTypeStr=fixdt(1,32,11)  AccumMin=[]  AccumMax=[]  InternalRndMeth=Nearest  InternalSaturateOnIntegerOverflow=off  SampleTime=-1
      settings: DataFormat=C
  head_in_cast : DataTypeConversion  OutDataTypeStr=fixdt(1,8,2)  RndMeth=Nearest
  head_out_cast : DataTypeConversion  OutDataTypeStr=single  SaturateOnIntegerOverflow=off  RndMeth=Floor
  patch_conv : dlconvfclib/Convolution 2D Layer  Layer=quantNet.Layers(2)  OutMin=[]  OutMax=[]  OutDataTypeStr=fixdt(1,32,12)  RndMeth=Nearest  SaturateOnIntegerOverflow=on  WeightsDataTypeStr=fixdt(1,8,8)  WeightsMin=[]  WeightsMax=[]  BiasDataTypeStr=fixdt(1,32,12)  BiasMin=[]  BiasMax=[]  AccumDataTypeStr=fixdt(1,32,12)  InternalRndMeth=Nearest  InternalSaturateOnIntegerOverflow=off  SampleTime=-1
      settings: DataFormat=SSC
  patch_conv_in_cast : DataTypeConversion  OutDataTypeStr=fixdt(1,8,4)  RndMeth=Nearest
  patch_conv_out_cast : DataTypeConversion  OutDataTypeStr=fixdt('single')  RndMeth=Nearest
  patch_flatten : Subsystem
  pos_embed : Subsystem
  head_out : Outport
  wires:
  block1_attn/1(out) -> block1_add1/1
  block1_ln1/1 -> block1_attn/1(in)
  block6_ln1/1 -> block6_attn/1(in)
  block5_ln1/1 -> block5_attn/1(in)
  block5_fc1/1 -> block5_fc1_out_cast/1
  patch_flatten/1(out) -> cls_prepend/1(in)
  block5_gelu/1 -> block5_fc2_in_cast/1
  block0_ln2/1 -> block0_fc1_in_cast/1
  block0_gelu/1 -> block0_fc2_in_cast/1
  block8_ln1/1 -> block8_attn/1(in)
  block0_fc1_out_cast/1 -> block0_gelu/1
  block5_fc2/1 -> block5_fc2_out_cast/1
  block2_fc1/1 -> block2_fc1_out_cast/1
  block6_fc1/1 -> block6_fc1_out_cast/1
  patch_conv_in_cast/1 -> patch_conv/1
  block8_fc2/1 -> block8_fc2_out_cast/1
  block1_ln2/1 -> block1_fc1_in_cast/1
  block2_fc2_in_cast/1 -> block2_fc2/1
  block11_fc1_out_cast/1 -> block11_gelu/1
  block9_fc2_out_cast/1 -> block9_add2/1
  block10_fc2_out_cast/1 -> block10_add2/1
  block1_fc2_in_cast/1 -> block1_fc2/1
  block10_ln2/1 -> block10_fc1_in_cast/1
  head_out_cast/1 -> head_out/1
  patch_conv_out_cast/1 -> patch_flatten/1(in)
  head/1 -> head_out_cast/1
  block3_attn/1(out) -> block3_add1/1
  head_in_cast/1 -> head/1
  block7_fc1_in_cast/1 -> block7_fc1/1
  block6_gelu/1 -> block6_fc2_in_cast/1
  block8_ln2/1 -> block8_fc1_in_cast/1
  block11_fc2_out_cast/1 -> block11_add2/1
  block7_fc2_out_cast/1 -> block7_add2/1
  block7_fc2/1 -> block7_fc2_out_cast/1
  block9_fc1_in_cast/1 -> block9_fc1/1
  block9_ln2/1 -> block9_fc1_in_cast/1
  block7_attn/1(out) -> block7_add1/1
  block3_fc1/1 -> block3_fc1_out_cast/1
  block2_gelu/1 -> block2_fc2_in_cast/1
  block5_fc1_out_cast/1 -> block5_gelu/1
  block2_ln1/1 -> block2_attn/1(in)
  block5_fc2_in_cast/1 -> block5_fc2/1
  block8_fc2_in_cast/1 -> block8_fc2/1
  block9_add2/1 -> block10_ln1/1, block10_add1/2
  patch_conv/1 -> patch_conv_out_cast/1
  block2_fc1_in_cast/1 -> block2_fc1/1
  block10_fc1/1 -> block10_fc1_out_cast/1
  block9_fc1/1 -> block9_fc1_out_cast/1
  block4_fc1/1 -> block4_fc1_out_cast/1
  block10_fc2/1 -> block10_fc2_out_cast/1
  block4_ln2/1 -> block4_fc1_in_cast/1
  block3_fc2/1 -> block3_fc2_out_cast/1
  block3_fc1_in_cast/1 -> block3_fc1/1
  block3_ln2/1 -> block3_fc1_in_cast/1
  block4_ln1/1 -> block4_attn/1(in)
  block11_add2/1 -> final_ln/1
  block10_gelu/1 -> block10_fc2_in_cast/1
  block3_gelu/1 -> block3_fc2_in_cast/1
  block9_fc2/1 -> block9_fc2_out_cast/1
  block6_fc2_out_cast/1 -> block6_add2/1
  block10_attn/1(out) -> block10_add1/1
  block7_add1/1 -> block7_add2/2, block7_ln2/1
  block9_attn/1(out) -> block9_add1/1
  block1_add1/1 -> block1_ln2/1, block1_add2/2
  block0_ln1/1 -> block0_attn/1(in)
  block5_ln2/1 -> block5_fc1_in_cast/1
  block10_fc1_out_cast/1 -> block10_gelu/1
  block11_attn/1(out) -> block11_add1/1
  block4_fc1_out_cast/1 -> block4_gelu/1
  block4_fc2_out_cast/1 -> block4_add2/1
  block1_fc2_out_cast/1 -> block1_add2/1
  block8_fc1/1 -> block8_fc1_out_cast/1
  block5_fc1_in_cast/1 -> block5_fc1/1
  block6_add2/1 -> block7_ln1/1, block7_add1/2
  block0_add2/1 -> block1_ln1/1, block1_add1/2
  block0_fc1_in_cast/1 -> block0_fc1/1
  block3_fc1_out_cast/1 -> block3_gelu/1
  block1_fc1/1 -> block1_fc1_out_cast/1
  block7_add2/1 -> block8_ln1/1, block8_add1/2
  block2_fc2/1 -> block2_fc2_out_cast/1
  block8_attn/1(out) -> block8_add1/1
  block8_gelu/1 -> block8_fc2_in_cast/1
  block1_fc2/1 -> block1_fc2_out_cast/1
  block1_gelu/1 -> block1_fc2_in_cast/1
  block0_fc1/1 -> block0_fc1_out_cast/1
  block4_add2/1 -> block5_ln1/1, block5_add1/2
  block1_add2/1 -> block2_add1/2, block2_ln1/1
  block6_fc2/1 -> block6_fc2_out_cast/1
  block10_add2/1 -> block11_ln1/1, block11_add1/2
  block8_fc2_out_cast/1 -> block8_add2/1
  block7_gelu/1 -> block7_fc2_in_cast/1
  block4_fc2/1 -> block4_fc2_out_cast/1
  block6_ln2/1 -> block6_fc1_in_cast/1
  pos_embed/1(out) -> block0_ln1/1, block0_add1/2
  block9_fc2_in_cast/1 -> block9_fc2/1
  input/1 -> patch_conv_in_cast/1
  block11_ln1/1 -> block11_attn/1(in)
  block3_ln1/1 -> block3_attn/1(in)
  block0_fc2/1 -> block0_fc2_out_cast/1
  block2_fc2_out_cast/1 -> block2_add2/1
  block7_fc1_out_cast/1 -> block7_gelu/1
  block11_fc1_in_cast/1 -> block11_fc1/1
  block4_fc2_in_cast/1 -> block4_fc2/1
  block6_fc1_out_cast/1 -> block6_gelu/1
  block7_ln2/1 -> block7_fc1_in_cast/1
  cls_extract/1(out) -> head_in_cast/1
  block9_gelu/1 -> block9_fc2_in_cast/1
  block6_attn/1(out) -> block6_add1/1
  final_ln/1 -> cls_extract/1(in)
  block4_gelu/1 -> block4_fc2_in_cast/1
  block9_add1/1 -> block9_add2/2, block9_ln2/1
  block8_add1/1 -> block8_ln2/1, block8_add2/2
  block4_add1/1 -> block4_ln2/1, block4_add2/2
  block0_fc2_out_cast/1 -> block0_add2/1
  block10_fc1_in_cast/1 -> block10_fc1/1
  block1_fc1_in_cast/1 -> block1_fc1/1
  block0_fc2_in_cast/1 -> block0_fc2/1
  block5_add1/1 -> block5_ln2/1, block5_add2/2
  block8_fc1_out_cast/1 -> block8_gelu/1
  block11_fc2_in_cast/1 -> block11_fc2/1
  block5_fc2_out_cast/1 -> block5_add2/1
  block9_fc1_out_cast/1 -> block9_gelu/1
  block11_fc1/1 -> block11_fc1_out_cast/1
  block10_add1/1 -> block10_ln2/1, block10_add2/2
  block4_attn/1(out) -> block4_add1/1
  block4_fc1_in_cast/1 -> block4_fc1/1
  block9_ln1/1 -> block9_attn/1(in)
  block3_add1/1 -> block3_ln2/1, block3_add2/2
  block2_add2/1 -> block3_ln1/1, block3_add1/2
  block3_fc2_in_cast/1 -> block3_fc2/1
  block5_attn/1(out) -> block5_add1/1
  block2_fc1_out_cast/1 -> block2_gelu/1
  block7_fc2_in_cast/1 -> block7_fc2/1
  block7_ln1/1 -> block7_attn/1(in)
  block3_fc2_out_cast/1 -> block3_add2/1
  block11_ln2/1 -> block11_fc1_in_cast/1
  block11_gelu/1 -> block11_fc2_in_cast/1
  block6_fc1_in_cast/1 -> block6_fc1/1
  block7_fc1/1 -> block7_fc1_out_cast/1
  cls_prepend/1(out) -> pos_embed/1(in)
  block1_fc1_out_cast/1 -> block1_gelu/1
  block10_ln1/1 -> block10_attn/1(in)
  block0_attn/1(out) -> block0_add1/1
  block11_add1/1 -> block11_ln2/1, block11_add2/2
  block0_add1/1 -> block0_ln2/1, block0_add2/2
  block8_fc1_in_cast/1 -> block8_fc1/1
  block10_fc2_in_cast/1 -> block10_fc2/1
  block6_add1/1 -> block6_ln2/1, block6_add2/2
  block2_ln2/1 -> block2_fc1_in_cast/1
  block2_add1/1 -> block2_ln2/1, block2_add2/2
  block3_add2/1 -> block4_ln1/1, block4_add1/2
  block6_fc2_in_cast/1 -> block6_fc2/1
  block2_attn/1(out) -> block2_add1/1
  block11_fc2/1 -> block11_fc2_out_cast/1
  block5_add2/1 -> block6_add1/2, block6_ln1/1
  block8_add2/1 -> block9_ln1/1, block9_add1/2

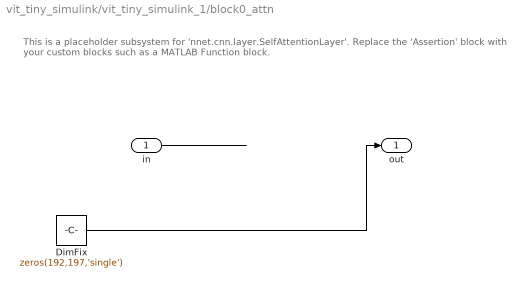
== system vit_tiny_simulink/vit_tiny_simulink_1/block0_attn ==
  note: This is a placeholder subsystem for 'nnet.cnn.layer.SelfAttentionLayer'. Replace the 'Assertion' block with your custom blocks such as a MATLAB Function block.
  in : Inport
  DimFix : Constant  Value=zeros(192,197,'single')  OutDataTypeStr=single  SampleTime=-1
  out : Outport
  wires:
  in/1 -> ?
  DimFix/1 -> out/1

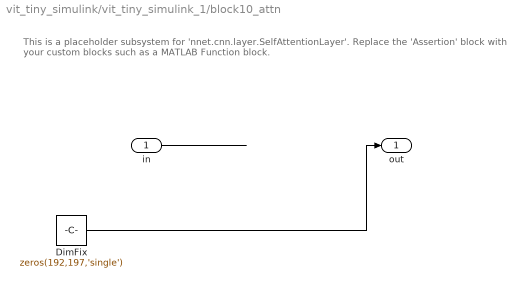
== system vit_tiny_simulink/vit_tiny_simulink_1/block10_attn ==
  note: This is a placeholder subsystem for 'nnet.cnn.layer.SelfAttentionLayer'. Replace the 'Assertion' block with your custom blocks such as a MATLAB Function block.
  in : Inport
  DimFix : Constant  Value=zeros(192,197,'single')  OutDataTypeStr=single  SampleTime=-1
  out : Outport
  wires:
  in/1 -> ?
  DimFix/1 -> out/1

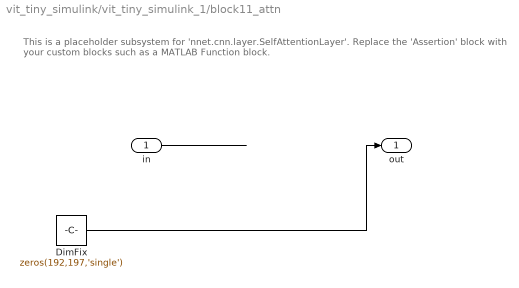
== system vit_tiny_simulink/vit_tiny_simulink_1/block11_attn ==
  note: This is a placeholder subsystem for 'nnet.cnn.layer.SelfAttentionLayer'. Replace the 'Assertion' block with your custom blocks such as a MATLAB Function block.
  in : Inport
  DimFix : Constant  Value=zeros(192,197,'single')  OutDataTypeStr=single  SampleTime=-1
  out : Outport
  wires:
  in/1 -> ?
  DimFix/1 -> out/1

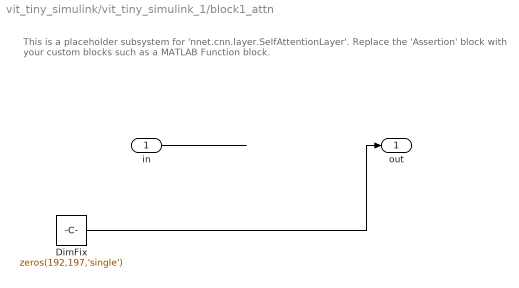
== system vit_tiny_simulink/vit_tiny_simulink_1/block1_attn ==
  note: This is a placeholder subsystem for 'nnet.cnn.layer.SelfAttentionLayer'. Replace the 'Assertion' block with your custom blocks such as a MATLAB Function block.
  in : Inport
  DimFix : Constant  Value=zeros(192,197,'single')  OutDataTypeStr=single  SampleTime=-1
  out : Outport
  wires:
  in/1 -> ?
  DimFix/1 -> out/1

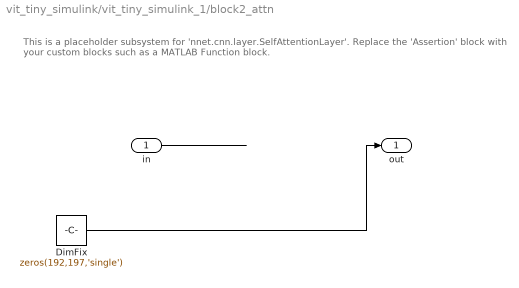
== system vit_tiny_simulink/vit_tiny_simulink_1/block2_attn ==
  note: This is a placeholder subsystem for 'nnet.cnn.layer.SelfAttentionLayer'. Replace the 'Assertion' block with your custom blocks such as a MATLAB Function block.
  in : Inport
  DimFix : Constant  Value=zeros(192,197,'single')  OutDataTypeStr=single  SampleTime=-1
  out : Outport
  wires:
  in/1 -> ?
  DimFix/1 -> out/1

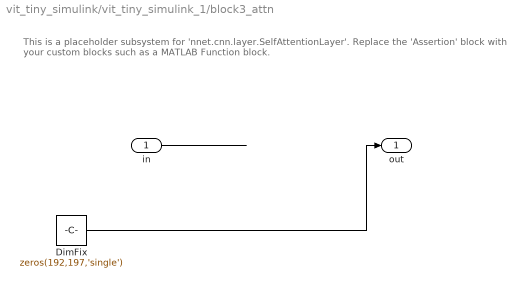
== system vit_tiny_simulink/vit_tiny_simulink_1/block3_attn ==
  note: This is a placeholder subsystem for 'nnet.cnn.layer.SelfAttentionLayer'. Replace the 'Assertion' block with your custom blocks such as a MATLAB Function block.
  in : Inport
  DimFix : Constant  Value=zeros(192,197,'single')  OutDataTypeStr=single  SampleTime=-1
  out : Outport
  wires:
  in/1 -> ?
  DimFix/1 -> out/1

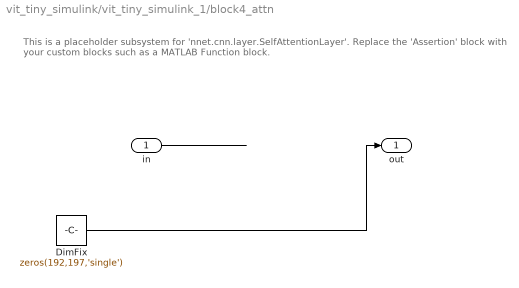
== system vit_tiny_simulink/vit_tiny_simulink_1/block4_attn ==
  note: This is a placeholder subsystem for 'nnet.cnn.layer.SelfAttentionLayer'. Replace the 'Assertion' block with your custom blocks such as a MATLAB Function block.
  in : Inport
  DimFix : Constant  Value=zeros(192,197,'single')  OutDataTypeStr=single  SampleTime=-1
  out : Outport
  wires:
  in/1 -> ?
  DimFix/1 -> out/1

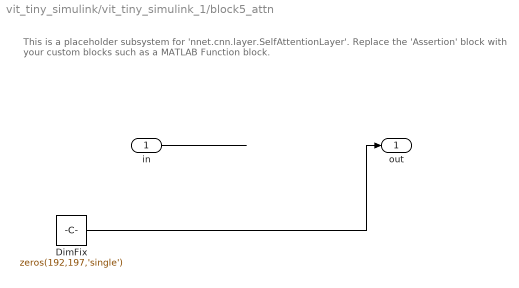
== system vit_tiny_simulink/vit_tiny_simulink_1/block5_attn ==
  note: This is a placeholder subsystem for 'nnet.cnn.layer.SelfAttentionLayer'. Replace the 'Assertion' block with your custom blocks such as a MATLAB Function block.
  in : Inport
  DimFix : Constant  Value=zeros(192,197,'single')  OutDataTypeStr=single  SampleTime=-1
  out : Outport
  wires:
  in/1 -> ?
  DimFix/1 -> out/1

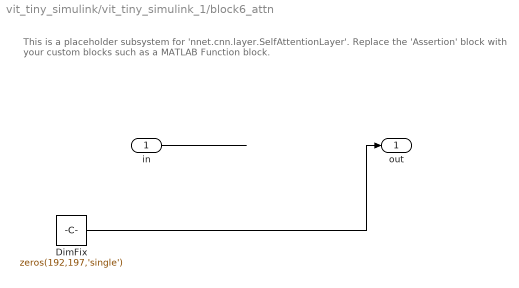
== system vit_tiny_simulink/vit_tiny_simulink_1/block6_attn ==
  note: This is a placeholder subsystem for 'nnet.cnn.layer.SelfAttentionLayer'. Replace the 'Assertion' block with your custom blocks such as a MATLAB Function block.
  in : Inport
  DimFix : Constant  Value=zeros(192,197,'single')  OutDataTypeStr=single  SampleTime=-1
  out : Outport
  wires:
  in/1 -> ?
  DimFix/1 -> out/1

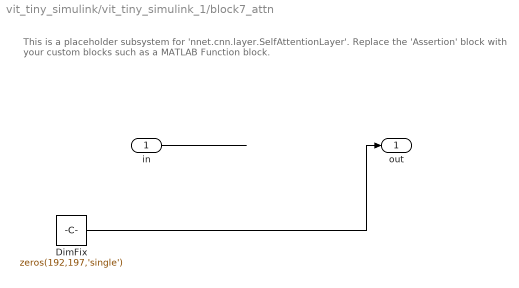
== system vit_tiny_simulink/vit_tiny_simulink_1/block7_attn ==
  note: This is a placeholder subsystem for 'nnet.cnn.layer.SelfAttentionLayer'. Replace the 'Assertion' block with your custom blocks such as a MATLAB Function block.
  in : Inport
  DimFix : Constant  Value=zeros(192,197,'single')  OutDataTypeStr=single  SampleTime=-1
  out : Outport
  wires:
  in/1 -> ?
  DimFix/1 -> out/1

== system vit_tiny_simulink/vit_tiny_simulink_1/block8_attn ==
  note: This is a placeholder subsystem for 'nnet.cnn.layer.SelfAttentionLayer'. Replace the 'Assertion' block with your custom blocks such as a MATLAB Function block.
  in : Inport
  DimFix : Constant  Value=zeros(192,197,'single')  OutDataTypeStr=single  SampleTime=-1
  out : Outport
  wires:
  in/1 -> ?
  DimFix/1 -> out/1

== system vit_tiny_simulink/vit_tiny_simulink_1/block9_attn ==
  note: This is a placeholder subsystem for 'nnet.cnn.layer.SelfAttentionLayer'. Replace the 'Assertion' block with your custom blocks such as a MATLAB Function block.
  in : Inport
  DimFix : Constant  Value=zeros(192,197,'single')  OutDataTypeStr=single  SampleTime=-1
  out : Outport
  wires:
  in/1 -> ?
  DimFix/1 -> out/1

== system vit_tiny_simulink/vit_tiny_simulink_1/cls_extract ==
  note: This is a placeholder subsystem for 'nnet.cnn.layer.Indexing1DLayer'. Replace the 'Assertion' block with your custom blocks such as a MATLAB Function block.
  in : Inport
  DimFix : Constant  Value=zeros(192,1,'single')  OutDataTypeStr=single  SampleTime=-1
  out : Outport
  wires:
  in/1 -> ?
  DimFix/1 -> out/1

== system vit_tiny_simulink/vit_tiny_simulink_1/cls_prepend ==
  note: This is a placeholder subsystem for 'nnet.cnn.layer.EmbeddingConcatenationLayer'. Replace the 'Assertion' block with your custom blocks such as a MATLAB Function block.
  in : Inport
  DimFix : Constant  Value=zeros(192,197,'single')  OutDataTypeStr=single  SampleTime=-1
  out : Outport
  wires:
  in/1 -> ?
  DimFix/1 -> out/1

== system vit_tiny_simulink/vit_tiny_simulink_1/patch_flatten ==
  note: This is a placeholder subsystem for 'PatchFlattenLayer'. Replace the 'Assertion' block with your custom blocks such as a MATLAB Function block.
  in : Inport
  DimFix : Constant  Value=zeros(192,196,'single')  OutDataTypeStr=single  SampleTime=-1
  out : Outport
  wires:
  in/1 -> ?
  DimFix/1 -> out/1

== system vit_tiny_simulink/vit_tiny_simulink_1/pos_embed ==
  note: This is a placeholder subsystem for 'AddPositionEmbeddingLayer'. Replace the 'Assertion' block with your custom blocks such as a MATLAB Function block.
  in : Inport
  DimFix : Constant  Value=zeros(192,197,'single')  OutDataTypeStr=single  SampleTime=-1
  out : Outport
  wires:
  in/1 -> ?
  DimFix/1 -> out/1
